simulink model "ident_2019b"  (R2019b)
settings: Solver=FixedStepAuto  StartTime=0.0  StopTime=20  FixedStep=Ts  RelTol=1e-3
values from neighbouring files (symbols this model uses):
  Flux = 0.00103001    [motor_parameters.sldd]
  Ld = 2.235E-5    [motor_parameters.sldd]
  Ls = 2.235E-5    [motor_parameters.sldd]
  Pn = 7.0    [motor_parameters.sldd]
  Rs = 0.112    [motor_parameters.sldd]
  Ts = 0.0001    [motor_parameters.sldd]
  Ubus = 12.0    [motor_parameters.sldd]
undefined symbols (not defined in the file or in its folder): magnitude
libraries: mcbplantlib x1, mcbcontrolslib x1, autolibpmsmexterior x1
settings Model: DataDictionary=motor_parameters.sldd  Creator=chenpeng  LastModifiedBy=ackict

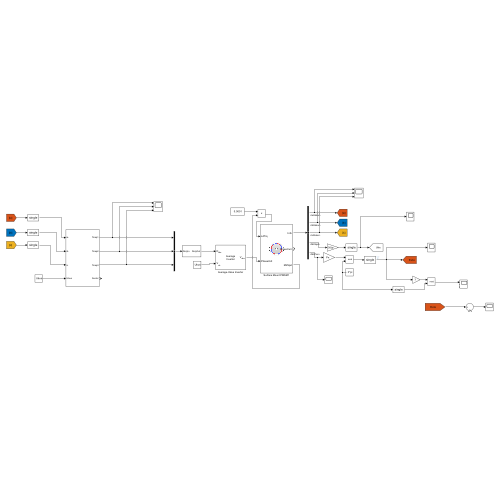
[thumbnail: Simulink's stored preview of the top-level diagram]
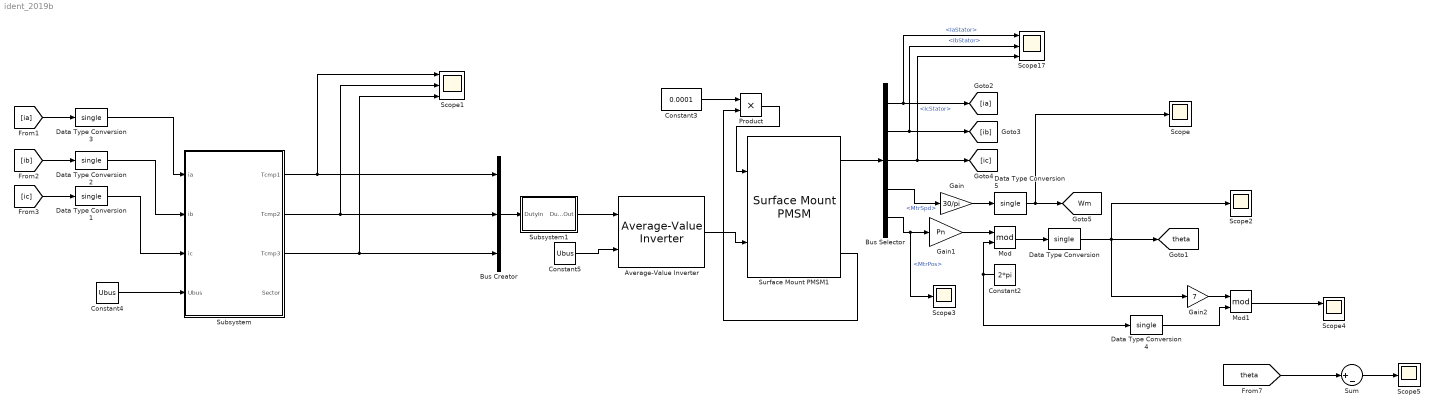
== system ident_2019b ==
  Average-Value Inverter : mcbplantlib/Average-Value Inverter
  Bus Creator : BusCreator  Inputs=3
  Bus Selector : BusSelector  OutputSignals=IaStator,IbStator,IcStator,MtrSpd,MtrPos
  Constant2 : Constant  Value=2*pi
  Constant3 : Constant  Value=0.0001  OutDataTypeStr=double
  Constant4 : Constant  Value=Ubus  OutDataTypeStr=single
  Constant5 : Constant  Value=Ubus  OutDataTypeStr=single
  Data Type Conversion{,1..5} (6 alike) : DataTypeConversion  OutDataTypeStr=single
  Gain : Gain  Gain=30/pi
  Gain1 : Gain  Gain=Pn
  Gain2 : Gain  Gain=7
  Mod : Math  Operator=mod  SaturateOnIntegerOverflow=on
  Mod1 : Math  Operator=mod  SaturateOnIntegerOverflow=on
  Product : Product
  Scope{,2..3,5} (4 alike) : Scope
  Scope1 : Scope  NumInputPorts=3
  Scope17 : Scope  NumInputPorts=3
  Scope4 : Scope  NumInputPorts=2
  Subsystem : Subsystem
  Subsystem1 : Subsystem
  Sum : Sum  Inputs=|+-
  Surface Mount PMSM1 : autolibpmsmexterior/Surface Mount PMSM  port_config=Torque  sim_type=Discrete  Ts=Ts  FilePath=E:\Sandbox\Bauto\Work\surfacepmsm_motordata.m  P=Pn  Rs=Rs  Ldq_=Ls  KConstText=Permanent flux linkage constant (lambda_pm):  lambda_pm=Flux  Ke=159.9771  Kt=1.323  mechanical=[0.0027, 4.924e-4, 0]  idq0=[0 0]  theta_init=0  omega_init=0  KConst=Flux  lambda_pm_calc=Flux  RefBlkName='autolibpmsmexterior/Surface Mount PMSM'  aMode=1  Ldq="[0.0003752   0.0003752]"
  tag scope: Wm=global, theta=global
  wires:
  Data Type Conversion3/1 -> Subsystem/1(ia)
  [ic] -> Data Type Conversion1/1
  Data Type Conversion1/1 -> Subsystem/3(ic)
  [ib] -> Data Type Conversion2/1
  [ia] -> Data Type Conversion3/1
  Data Type Conversion2/1 -> Subsystem/2(ib)
  Constant4/1 -> Subsystem/4(Ubus)
  Mod/1 -> Data Type Conversion/1
  Bus Selector/2 -> Scope17/2, [ib]  "<IbStator>"
  Subsystem/3(Tcmp3) -> Scope1/3, Bus Creator/3
  Data Type Conversion4/1 -> Mod1/2
  Constant2/1 -> Data Type Conversion4/1, Mod/2
  Subsystem/1(Tcmp1) -> Bus Creator/1, Scope1/1
  [theta] -> Sum/1
  Sum/1 -> Scope5/1
  Subsystem/2(Tcmp2) -> Scope1/2, Bus Creator/2
  Bus Selector/4 -> Gain/1  "<MtrSpd>"
  Product/1 -> Surface Mount PMSM1/1
  Mod1/1 -> Scope4/1
  Surface Mount PMSM1/1 -> Bus Selector/1
  Gain2/1 -> Mod1/1
  Surface Mount PMSM1/3 -> Product/2
  Subsystem1/1(DutyOut) -> Average-Value Inverter/1
  Constant5/1 -> Average-Value Inverter/2
  Average-Value Inverter/1 -> Surface Mount PMSM1/2
  Bus Selector/1 -> [ia], Scope17/1  "<IaStator>"
  Bus Selector/5 -> Scope3/1, Gain1/1  "<MtrPos>"
  Bus Creator/1 -> Subsystem1/1(DutyIn)
  Data Type Conversion/1 -> Scope2/1, Gain2/1, [theta]
  Bus Selector/3 -> Scope17/3, [ic]  "<IcStator>"
  Gain1/1 -> Mod/1
  Constant3/1 -> Product/1
  Data Type Conversion5/1 -> Scope/1, [Wm]
  Gain/1 -> Data Type Conversion5/1

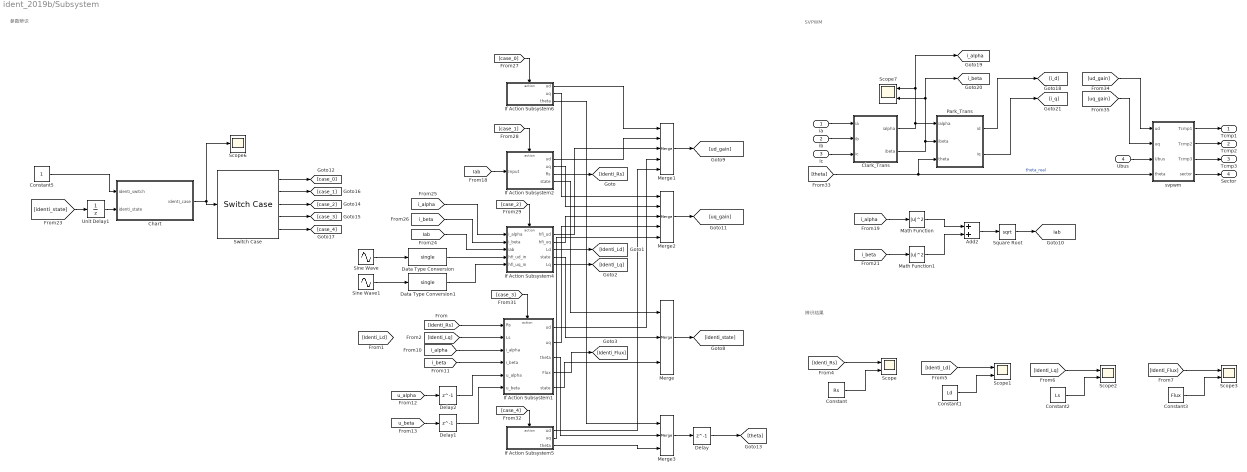
== system ident_2019b/Subsystem ==
  note: 参数辨识
  note: 辨识结果
  note: SVPWM
  ia : Inport  OutDataTypeStr=single  SampleTime=0.0001
  ib : Inport  Port=2  OutDataTypeStr=single  SampleTime=0.0001
  ic : Inport  Port=3  OutDataTypeStr=single  SampleTime=0.0001
  Ubus : Inport  Port=4  SampleTime=0.0001
  Add2 : Sum
  Chart : Stateflow chart  TreatAsAtomicUnit=on
  Clark_Trans : Subsystem  TreatAsAtomicUnit=on
  Constant : Constant  Value=Rs  OutDataTypeStr=single
  Constant1 : Constant  Value=Ld  OutDataTypeStr=single
  Constant2 : Constant  Value=Ls  OutDataTypeStr=single
  Constant3 : Constant  Value=Flux  OutDataTypeStr=single
  Constant5 : Constant  OutDataTypeStr=single
  Data Type Conversion : DataTypeConversion  OutDataTypeStr=single
  Data Type Conversion1 : DataTypeConversion  OutDataTypeStr=single
  Delay : Delay  DelayLength=1
  Delay1 : Delay  DelayLength=1
  Delay2 : Delay  DelayLength=1
  If Action Subsystem1 : Subsystem  TreatAsAtomicUnit=on
  If Action Subsystem2 : Subsystem  TreatAsAtomicUnit=on
  If Action Subsystem4 : Subsystem  TreatAsAtomicUnit=on
  If Action Subsystem5 : Subsystem  TreatAsAtomicUnit=on
  If Action Subsystem6 : Subsystem  TreatAsAtomicUnit=on
  Math Function : Math  Operator=magnitude^2  SignedPower=on  OutputSignalType=real  SaturateOnIntegerOverflow=on
  Math Function1 : Math  Operator=magnitude^2  SignedPower=on  OutputSignalType=real  SaturateOnIntegerOverflow=on
  Merge : Merge  Inputs=3
  Merge1 : Merge  Inputs=5
  Merge2 : Merge  Inputs=5
  Merge3 : Merge  Inputs=3
  Park_Trans : Subsystem  TreatAsAtomicUnit=on
  Scope{,1..3,7} (5 alike) : Scope  NumInputPorts=2
  Scope6 : Scope
  Sine Wave : Sin  Amplitude=2  Frequency=1884  SampleTime=0.0001
  Sine Wave1 : Sin  Amplitude=2  Frequency=1884  Phase=pi/2  SampleTime=0.0001
  Square Root : Sqrt  SaturateOnIntegerOverflow=on
  Switch Case : SwitchCase  CaseConditions={0,1,2,3,4}  ShowDefaultCase=off
  Unit Delay1 : UnitDelay  SampleTime=-1  HasFrameUpgradeWarning=on
  svpwm : Subsystem
  Tcmp1 : Outport
  Tcmp2 : Outport  Port=2
  Tcmp3 : Outport  Port=3
  Sector : Outport  Port=4
  tag scope: Iab=global, i_alpha=global, i_beta=global
  wires:
  If Action Subsystem6/1(ud) -> Merge1/1
  Data Type Conversion1/1 -> If Action Subsystem4/5(hfi_uq_in)
  Switch Case/1 -> [case_0]
  If Action Subsystem1/4(Flux) -> [Identi_Flux]
  If Action Subsystem4/2(hfi_uq) -> Merge2/3
  Merge/1 -> [identi_state]
  Ubus/1 -> svpwm/3(Ubus)
  Clark_Trans/2(ibeta) -> [i_beta], Scope7/2, Park_Trans/2(ibeta)
  If Action Subsystem4/4(state) -> Merge/2
  Switch Case/4 -> [case_3]
  If Action Subsystem2/2(uq) -> Merge2/2
  Clark_Trans/1(ialpha) -> [i_alpha], Scope7/1, Park_Trans/1(ialpha)
  Switch Case/2 -> [case_1]
  Merge3/1 -> Delay/1
  Math Function1/1 -> Add2/2
  [i_beta] -> If Action Subsystem4/2(i_beta)
  [theta] -> svpwm/4(theta), Park_Trans/3(theta)  "theta_real"
  [Iab] -> If Action Subsystem4/3(iab)
  If Action Subsystem6/3(theta) -> Merge3/1
  [ud_gain] -> svpwm/1(ud)
  Data Type Conversion/1 -> If Action Subsystem4/4(hfi_ud_in)
  If Action Subsystem5/2(uq) -> Merge2/5
  svpwm/4(sector) -> Sector/1
  Park_Trans/2(iq) -> [i_q]
  [case_3] -> If Action Subsystem1/Action
  Sine Wave/1 -> Data Type Conversion/1
  If Action Subsystem2/1(ud) -> Merge1/2
  Switch Case/3 -> [case_2]
  svpwm/1(Tcmp1) -> Tcmp1/1
  Constant5/1 -> Chart/1(identi_switch)
  [case_1] -> If Action Subsystem2/Action
  ia/1 -> Clark_Trans/1(ia)
  ic/1 -> Clark_Trans/3(ic)
  If Action Subsystem1/2(uq) -> Merge2/4
  [i_alpha] -> Math Function/1
  Math Function/1 -> Add2/1
  ib/1 -> Clark_Trans/2(ib)
  If Action Subsystem1/1(ud) -> Merge1/4
  If Action Subsystem5/3(theta) -> Merge3/3
  Square Root/1 -> [Iab]
  [case_4] -> If Action Subsystem5/Action
  Park_Trans/1(id) -> [i_d]
  Add2/1 -> Square Root/1
  [i_alpha] -> If Action Subsystem4/1(i_alpha)
  [Iab] -> If Action Subsystem2/1(Input)
  If Action Subsystem1/3(theta) -> Merge3/2
  Chart/1(identi_case) -> Scope6/1, Switch Case/1
  [case_0] -> If Action Subsystem6/Action
  [Identi_Lq] -> If Action Subsystem1/2(Ls)
  Switch Case/5 -> [case_4]
  [case_2] -> If Action Subsystem4/Action
  [i_beta] -> Math Function1/1
  Unit Delay1/1 -> Chart/2(identi_state)
  [identi_state] -> Unit Delay1/1
  Merge1/1 -> [ud_gain]
  Sine Wave1/1 -> Data Type Conversion1/1
  If Action Subsystem4/1(hfi_ud) -> Merge1/3
  svpwm/2(Tcmp2) -> Tcmp2/1
  svpwm/3(Tcmp3) -> Tcmp3/1
  Merge2/1 -> [uq_gain]
  If Action Subsystem5/1(ud) -> Merge1/5
  [uq_gain] -> svpwm/2(uq)
  If Action Subsystem2/4(state) -> Merge/1
  If Action Subsystem1/5(state) -> Merge/3
  If Action Subsystem6/2(uq) -> Merge2/1
  If Action Subsystem4/3(Ld) -> [Identi_Ld]
  [Identi_Rs] -> If Action Subsystem1/1(Rs)
  If Action Subsystem2/3(Rs) -> [Identi_Rs]
  [Identi_Rs] -> Scope/1
  Constant/1 -> Scope/2
  [Identi_Ld] -> Scope1/1
  Constant1/1 -> Scope1/2
  [Identi_Lq] -> Scope2/1
  Constant2/1 -> Scope2/2
  [Identi_Flux] -> Scope3/1
  Constant3/1 -> Scope3/2
  If Action Subsystem4/5(Lq) -> [Identi_Lq]
  [i_alpha] -> If Action Subsystem1/3(i_alpha)
  [i_beta] -> If Action Subsystem1/4(i_beta)
  Delay/1 -> [theta]
  Delay2/1 -> If Action Subsystem1/5(u_alpha)
  [u_alpha] -> Delay2/1
  [u_beta] -> Delay1/1
  Delay1/1 -> If Action Subsystem1/6(u_beta)

== system ident_2019b/Subsystem1 ==
  DutyIn : Inport
  Constant : Constant  Value=0.5  OutDataTypeStr=double  SampleTime=-1
  Gain : Gain  Gain=1/8000  ParamDataTypeStr=single
  Gain1 : Gain  Gain=-1
  Sum : Sum  Inputs=|+-
  Sum1 : Sum  Inputs=|++
  DutyOut : Outport
  wires:
  Sum/1 -> Gain1/1
  Constant/1 -> Sum1/2, Sum/2
  DutyIn/1 -> Gain/1
  Gain1/1 -> Sum1/1
  Sum1/1 -> DutyOut/1
  Gain/1 -> Sum/1

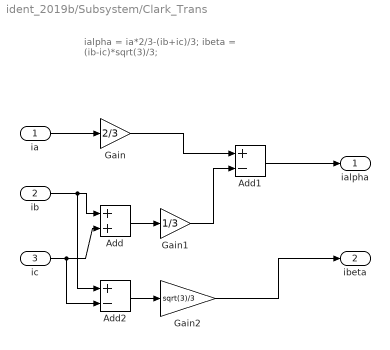
== system ident_2019b/Subsystem/Clark_Trans ==
  note: ialpha = ia*2/3-(ib+ic)/3;
      | ibeta = (ib-ic)*sqrt(3)/3;
  ia : Inport  OutDataTypeStr=single
  ib : Inport  Port=2  OutDataTypeStr=single
  ic : Inport  Port=3  OutDataTypeStr=single
  Add : Sum  AccumDataTypeStr=single  OutDataTypeStr=single
  Add1 : Sum  Inputs=+-  AccumDataTypeStr=single  OutDataTypeStr=single
  Add2 : Sum  Inputs=+-  AccumDataTypeStr=single  OutDataTypeStr=single
  Gain : Gain  Gain=2/3  ParamDataTypeStr=single
  Gain1 : Gain  Gain=1/3  ParamDataTypeStr=single
  Gain2 : Gain  Gain=sqrt(3)/3  ParamDataTypeStr=single
  ialpha : Outport  OutDataTypeStr=single
  ibeta : Outport  Port=2  OutDataTypeStr=single
  wires:
  ia/1 -> Gain/1
  ib/1 -> Add2/1, Add/1
  ic/1 -> Add2/2, Add/2
  Add/1 -> Gain1/1
  Gain/1 -> Add1/1
  Gain1/1 -> Add1/2
  Add1/1 -> ialpha/1
  Add2/1 -> Gain2/1
  Gain2/1 -> ibeta/1

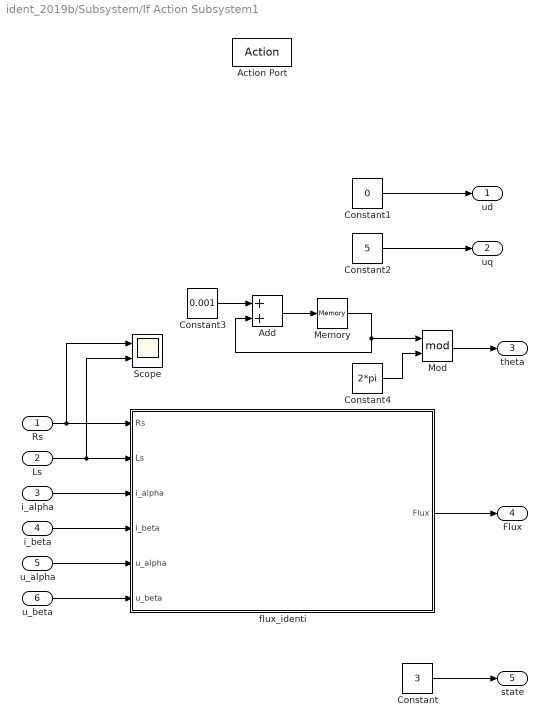
== system ident_2019b/Subsystem/If Action Subsystem1 ==
  Rs : Inport  OutDataTypeStr=single
  Ls : Inport  Port=2  OutDataTypeStr=single
  i_alpha : Inport  Port=3  OutDataTypeStr=single
  i_beta : Inport  Port=4  OutDataTypeStr=single
  u_alpha : Inport  Port=5  OutDataTypeStr=single
  u_beta : Inport  Port=6  OutDataTypeStr=single
  Action Port : ActionPort  ActionPortLabel=case [ 3 ]:
  Add : Sum
  Constant : Constant  Value=3  OutDataTypeStr=single
  Constant1 : Constant  Value=0  OutDataTypeStr=single
  Constant2 : Constant  Value=5  OutDataTypeStr=single
  Constant3 : Constant  Value=0.001  OutDataTypeStr=single
  Constant4 : Constant  Value=2*pi  OutDataTypeStr=single
  Memory : Memory
  Mod : Math  Operator=mod  SaturateOnIntegerOverflow=on
  Scope : Scope  NumInputPorts=2
  flux_identi : Subsystem
  ud : Outport  OutDataTypeStr=single
  uq : Outport  Port=2  OutDataTypeStr=single
  theta : Outport  Port=3  OutDataTypeStr=single
  Flux : Outport  Port=4  OutDataTypeStr=single
  state : Outport  Port=5  OutDataTypeStr=single
  wires:
  Constant/1 -> state/1
  Rs/1 -> Scope/1, flux_identi/1(Rs)
  Ls/1 -> Scope/2, flux_identi/2(Ls)
  flux_identi/1(Flux) -> Flux/1
  i_alpha/1 -> flux_identi/3(i_alpha)
  i_beta/1 -> flux_identi/4(i_beta)
  u_alpha/1 -> flux_identi/5(u_alpha)
  u_beta/1 -> flux_identi/6(u_beta)
  Constant1/1 -> ud/1
  Constant2/1 -> uq/1
  Constant3/1 -> Add/1
  Add/1 -> Memory/1
  Memory/1 -> Mod/1, Add/2
  Constant4/1 -> Mod/2
  Mod/1 -> theta/1

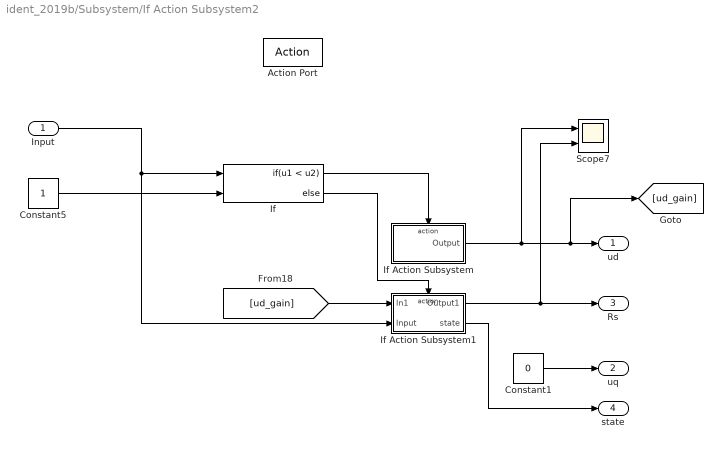
== system ident_2019b/Subsystem/If Action Subsystem2 ==
  Input : Inport  OutDataTypeStr=single
  Action Port : ActionPort  ActionPortLabel=case [ 1 ]:
  Constant1 : Constant  Value=0  OutDataTypeStr=single
  Constant5 : Constant  OutDataTypeStr=single
  If : If  NumInputs=2  IfExpression=u1 < u2
  If Action Subsystem : Subsystem  TreatAsAtomicUnit=on
  If Action Subsystem1 : Subsystem  TreatAsAtomicUnit=on
  Scope7 : Scope  NumInputPorts=2
  ud : Outport  OutDataTypeStr=single
  uq : Outport  Port=2  OutDataTypeStr=single
  Rs : Outport  Port=3  OutDataTypeStr=single
  state : Outport  Port=4  OutDataTypeStr=single
  wires:
  [ud_gain] -> If Action Subsystem1/1(In1)
  If/1 -> If Action Subsystem/Action
  If Action Subsystem/1(Output) -> Scope7/1, [ud_gain], ud/1
  Constant5/1 -> If/2
  If/2 -> If Action Subsystem1/Action
  Input/1 -> If Action Subsystem1/2(Input), If/1
  If Action Subsystem1/1(Output1) -> Rs/1, Scope7/2
  Constant1/1 -> uq/1
  If Action Subsystem1/2(state) -> state/1

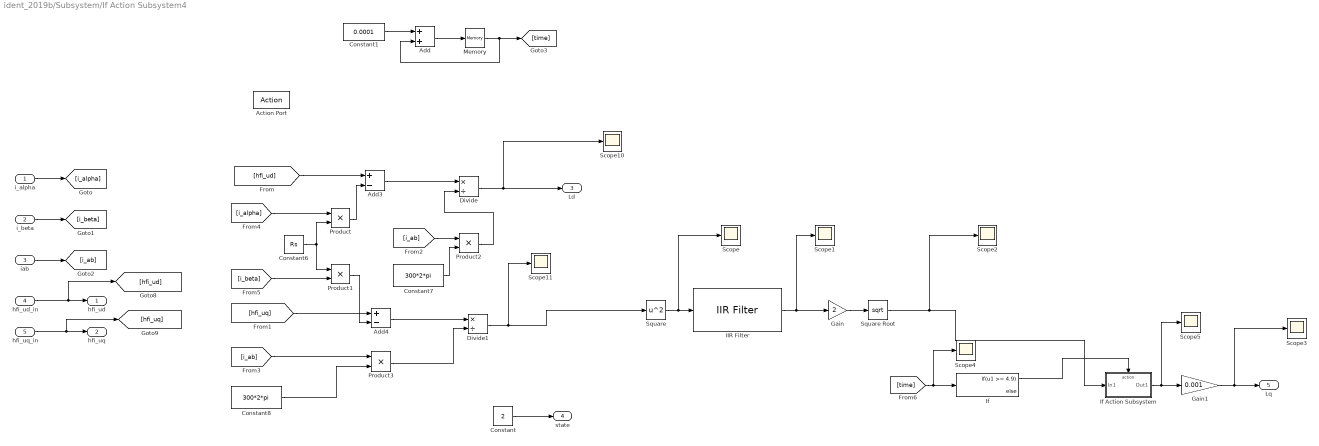
== system ident_2019b/Subsystem/If Action Subsystem4 ==
  i_alpha : Inport  OutDataTypeStr=single
  i_beta : Inport  Port=2  OutDataTypeStr=single
  iab : Inport  Port=3  OutDataTypeStr=single
  hfi_ud_in : Inport  Port=4  OutDataTypeStr=single
  hfi_uq_in : Inport  Port=5  OutDataTypeStr=single
  Action Port : ActionPort  ActionPortLabel=case [ 2 ]:
  Add : Sum
  Add3 : Sum  Inputs=+-  OutDataTypeStr=single
  Add4 : Sum  Inputs=+-  OutDataTypeStr=single
  Constant : Constant  Value=2  OutDataTypeStr=single
  Constant1 : Constant  Value=0.0001  OutDataTypeStr=single
  Constant6 : Constant  Value=Rs  OutDataTypeStr=single
  Constant7 : Constant  Value=300*2*pi  OutDataTypeStr=single
  Constant8 : Constant  Value=300*2*pi  OutDataTypeStr=single
  Divide : Product  Inputs=*/  OutDataTypeStr=single
  Divide1 : Product  Inputs=*/
  Gain : Gain  Gain=2
  Gain1 : Gain  Gain=0.001
  IIR Filter : mcbcontrolslib/IIR Filter  VariantControl=Low Pass Filter  VariantSelect=Low-pass  Filter_constant=0.0063  advancedSettings=on  Ts=1e-4  cutOff_freq=10.0903
  If : If  IfExpression=u1 >= 4.9
  If Action Subsystem : Subsystem  TreatAsAtomicUnit=on
  Memory : Memory
  Product : Product  OutDataTypeStr=single
  Product1 : Product  OutDataTypeStr=single
  Product2 : Product  OutDataTypeStr=single
  Product3 : Product
  Scope{,1..5,10..11} (8 alike) : Scope
  Square : Math  Operator=square  SaturateOnIntegerOverflow=on
  Square Root : Sqrt  OutDataTypeStr=single  SaturateOnIntegerOverflow=on
  hfi_ud : Outport  OutDataTypeStr=single
  hfi_uq : Outport  Port=2  OutDataTypeStr=single
  Ld : Outport  Port=3  OutDataTypeStr=single
  state : Outport  Port=4  OutDataTypeStr=single
  Lq : Outport  Port=5  OutDataTypeStr=single
  wires:
  Product/1 -> Add3/2
  Constant8/1 -> Product3/2
  Product3/1 -> Divide1/2
  Divide1/1 -> Square/1, Scope11/1
  [i_ab] -> Product3/1
  [hfi_uq] -> Add4/1
  Divide/1 -> Ld/1, Scope10/1
  [i_ab] -> Product2/1
  Product1/1 -> Add4/2
  Product2/1 -> Divide/2
  Add4/1 -> Divide1/1
  Constant7/1 -> Product2/2
  [hfi_ud] -> Add3/1
  Constant6/1 -> Product1/1, Product/2
  Add3/1 -> Divide/1
  [i_beta] -> Product1/2
  [i_alpha] -> Product/1
  Constant/1 -> state/1
  i_alpha/1 -> [i_alpha]
  i_beta/1 -> [i_beta]
  iab/1 -> [i_ab]
  hfi_uq_in/1 -> [hfi_uq], hfi_uq/1
  hfi_ud_in/1 -> [hfi_ud], hfi_ud/1
  Gain/1 -> Square Root/1
  Square/1 -> Scope/1, IIR Filter/1
  IIR Filter/1 -> Scope1/1, Gain/1
  Square Root/1 -> Scope2/1, If Action Subsystem/1(In1)
  Constant1/1 -> Add/1
  Add/1 -> Memory/1
  Memory/1 -> Add/2, [time]
  [time] -> Scope4/1, If/1
  If/1 -> If Action Subsystem/Action
  If Action Subsystem/1(Out1) -> Scope5/1, Gain1/1
  Gain1/1 -> Lq/1, Scope3/1

== system ident_2019b/Subsystem/If Action Subsystem5 ==
  Action Port : ActionPort  ActionPortLabel=case [ 4 ]:
  Constant : Constant  Value=0  OutDataTypeStr=single
  Constant1 : Constant  Value=0  OutDataTypeStr=single
  Constant2 : Constant  Value=0  OutDataTypeStr=single
  ud : Outport
  uq : Outport  Port=2  OutDataTypeStr=single
  theta : Outport  Port=3
  wires:
  Constant/1 -> uq/1
  Constant1/1 -> ud/1
  Constant2/1 -> theta/1

== system ident_2019b/Subsystem/If Action Subsystem6 ==
  Action Port : ActionPort  ActionPortLabel=case [ 0 ]:
  Constant : Constant  Value=0  OutDataTypeStr=single
  Constant1 : Constant  Value=0  OutDataTypeStr=single
  Constant2 : Constant  Value=0  OutDataTypeStr=single
  ud : Outport
  uq : Outport  Port=2  OutDataTypeStr=single
  theta : Outport  Port=3
  wires:
  Constant2/1 -> theta/1
  Constant1/1 -> ud/1
  Constant/1 -> uq/1

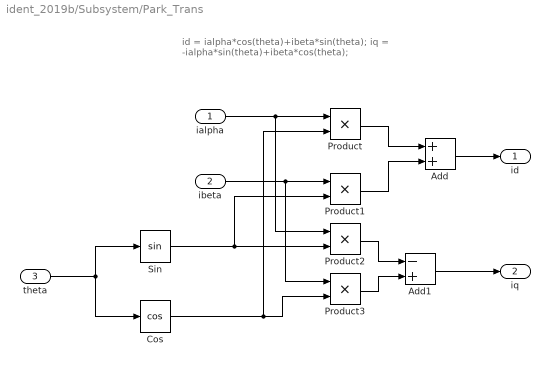
== system ident_2019b/Subsystem/Park_Trans ==
  note: id = ialpha*cos(theta)+ibeta*sin(theta);
      | iq = -ialpha*sin(theta)+ibeta*cos(theta);
  ialpha : Inport  OutDataTypeStr=single
  ibeta : Inport  Port=2  OutDataTypeStr=single
  theta : Inport  Port=3  OutDataTypeStr=single
  Add : Sum  AccumDataTypeStr=single  OutDataTypeStr=single
  Add1 : Sum  Inputs=-+  AccumDataTypeStr=single  OutDataTypeStr=single
  Cos : Trigonometry  Operator=cos  ApproximationMethod=CORDIC
  Product{,1..3} (4 alike) : Product  OutDataTypeStr=single
  Sin : Trigonometry  ApproximationMethod=CORDIC
  id : Outport  OutDataTypeStr=single
  iq : Outport  Port=2  OutDataTypeStr=single
  wires:
  ialpha/1 -> Product2/1, Product/1
  ibeta/1 -> Product3/1, Product1/1
  Product/1 -> Add/1
  Product1/1 -> Add/2
  Add/1 -> id/1
  Product2/1 -> Add1/1
  Product3/1 -> Add1/2
  Add1/1 -> iq/1
  theta/1 -> Cos/1, Sin/1
  Sin/1 -> Product1/2, Product2/2
  Cos/1 -> Product/2, Product3/2

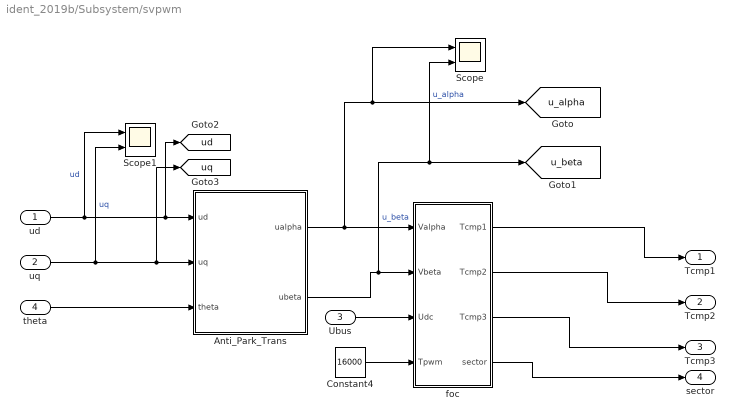
== system ident_2019b/Subsystem/svpwm ==
  ud : Inport  OutDataTypeStr=single
  uq : Inport  Port=2
  Ubus : Inport  Port=3  SampleTime=0.0001
  theta : Inport  Port=4
  Anti_Park_Trans : Subsystem  TreatAsAtomicUnit=on
  Constant4 : Constant  Value=16000  OutDataTypeStr=single
  Scope : Scope  NumInputPorts=2
  Scope1 : Scope  NumInputPorts=2
  foc : MATLAB Function  TreatAsAtomicUnit=on
  Tcmp1 : Outport
  Tcmp2 : Outport  Port=2
  Tcmp3 : Outport  Port=3
  sector : Outport  Port=4
  tag scope: u_alpha=global, u_beta=global, ud=global, uq=global
  wires:
  foc/1(Tcmp1) -> Tcmp1/1
  Constant4/1 -> foc/4(Tpwm)
  Ubus/1 -> foc/3(Udc)
  uq/1 -> Scope1/2, [uq], Anti_Park_Trans/2(uq)  "uq"
  foc/4(sector) -> sector/1
  ud/1 -> Scope1/1, [ud], Anti_Park_Trans/1(ud)  "ud"
  foc/3(Tcmp3) -> Tcmp3/1
  foc/2(Tcmp2) -> Tcmp2/1
  theta/1 -> Anti_Park_Trans/3(theta)
  Anti_Park_Trans/1(ualpha) -> Scope/1, [u_alpha], foc/1(Valpha)  "u_alpha"
  Anti_Park_Trans/2(ubeta) -> Scope/2, [u_beta], foc/2(Vbeta)  "u_beta"

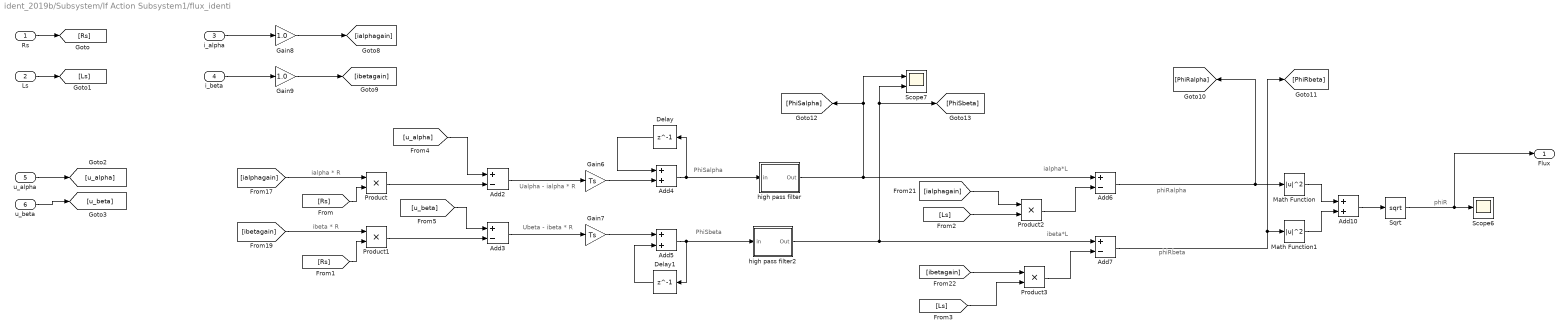
== system ident_2019b/Subsystem/If Action Subsystem1/flux_identi ==
  note: phiRbeta
  note: phiR
  note: ialpha * R
  note: PhiSbeta
  note: phiRalpha
  note: ialpha*L
  note: ibeta * R
  note: Ubeta - ibeta * R
  note: Ualpha - ialpha * R
  note: PhiSalpha
  note: ibeta*L
  Rs : Inport  OutDataTypeStr=single
  Ls : Inport  Port=2  OutDataTypeStr=single
  i_alpha : Inport  Port=3  OutDataTypeStr=single
  i_beta : Inport  Port=4  OutDataTypeStr=single
  u_alpha : Inport  Port=5  OutDataTypeStr=single
  u_beta : Inport  Port=6  OutDataTypeStr=single
  Add10 : Sum
  Add{2..3,6..7} (4 alike) : Sum  Inputs=+-
  Add4 : Sum
  Add5 : Sum
  Delay : Delay  DelayLength=1  InitialCondition=0
  Delay1 : Delay  DelayLength=1
  Gain6 : Gain  Gain=Ts
  Gain7 : Gain  Gain=Ts
  Gain8 : Gain  Gain=1.0
  Gain9 : Gain  Gain=1.0
  Math Function : Math  Operator=magnitude^2  SignedPower=on  OutputSignalType=real  SaturateOnIntegerOverflow=on
  Math Function1 : Math  Operator=magnitude^2  SignedPower=on  OutputSignalType=real  SaturateOnIntegerOverflow=on
  Product{,1..3} (4 alike) : Product
  Scope6 : Scope
  Scope7 : Scope  NumInputPorts=2
  Sqrt : Sqrt  SaturateOnIntegerOverflow=on
  high pass filter : Subsystem  mask{fc=10, Ts=Ts}
      mask prompts: fc "cut off freq"; Ts "simple rate"
      mask help: High pass filter
  high pass filter2 : Subsystem  mask{fc=10, Ts=Ts}
      mask prompts: fc "cut off freq"; Ts "simple rate"
      mask help: High pass filter
  Flux : Outport  OutDataTypeStr=single
  wires:
  Math Function1/1 -> Add10/2
  [u_beta] -> Add3/1
  Add6/1 -> [PhiRalpha], Math Function/1
  Add3/1 -> Gain7/1
  [ibetagain] -> Product3/1
  Add5/1 -> Delay1/1, high pass filter2/1(in)
  Add4/1 -> Delay/1, high pass filter/1(in)
  high pass filter/1(Out) -> [PhiSalpha], Scope7/1, Add6/1
  Gain6/1 -> Add4/2
  [ibetagain] -> Product1/1
  Add10/1 -> Sqrt/1
  Delay1/1 -> Add5/2
  [ialphagain] -> Product/1
  Math Function/1 -> Add10/1
  [u_alpha] -> Add2/1
  Product/1 -> Add2/2
  Product3/1 -> Add7/2
  Delay/1 -> Add4/1
  Add2/1 -> Gain6/1
  Sqrt/1 -> Flux/1, Scope6/1
  Product1/1 -> Add3/2
  i_beta/1 -> Gain9/1
  Add7/1 -> [PhiRbeta], Math Function1/1
  Gain7/1 -> Add5/1
  i_alpha/1 -> Gain8/1
  high pass filter2/1(Out) -> [PhiSbeta], Scope7/2, Add7/1
  Gain9/1 -> [ibetagain]
  Gain8/1 -> [ialphagain]
  Rs/1 -> [Rs]
  Ls/1 -> [Ls]
  [Rs] -> Product/2
  [Rs] -> Product1/2
  [ialphagain] -> Product2/1
  Product2/1 -> Add6/2
  [Ls] -> Product2/2
  [Ls] -> Product3/2
  u_alpha/1 -> [u_alpha]
  u_beta/1 -> [u_beta]

== system ident_2019b/Subsystem/If Action Subsystem2/If Action Subsystem ==
  Action Port : ActionPort  ActionPortLabel=if(u1 < u2)
  Add3 : Sum
  Constant6 : Constant  Value=0.01  OutDataTypeStr=single
  Memory : Memory  InheritSampleTime=on
  Output : Outport  OutDataTypeStr=single
  wires:
  Memory/1 -> Output/1, Add3/2
  Add3/1 -> Memory/1
  Constant6/1 -> Add3/1

== system ident_2019b/Subsystem/If Action Subsystem2/If Action Subsystem1 ==
  In1 : Inport  OutDataTypeStr=single
  Input : Inport  Port=2  OutDataTypeStr=single
  Action Port : ActionPort  ActionPortLabel=else
  Constant : Constant  OutDataTypeStr=single
  Divide : Product  Inputs=*/
  Output1 : Outport  OutDataTypeStr=single
  state : Outport  Port=2  OutDataTypeStr=single
  wires:
  In1/1 -> Divide/1
  Input/1 -> Divide/2
  Divide/1 -> Output1/1
  Constant/1 -> state/1

== system ident_2019b/Subsystem/If Action Subsystem4/If Action Subsystem ==
  In1 : Inport  OutDataTypeStr=single
  Action Port : ActionPort  ActionPortLabel=if(u1 >= 4.9)
  Memory : Memory
  Scope : Scope
  Sum : Sum  Inputs=|++
  Out1 : Outport  OutDataTypeStr=single
  wires:
  In1/1 -> Scope/1, Sum/1
  Sum/1 -> Memory/1
  Memory/1 -> Out1/1, Sum/2

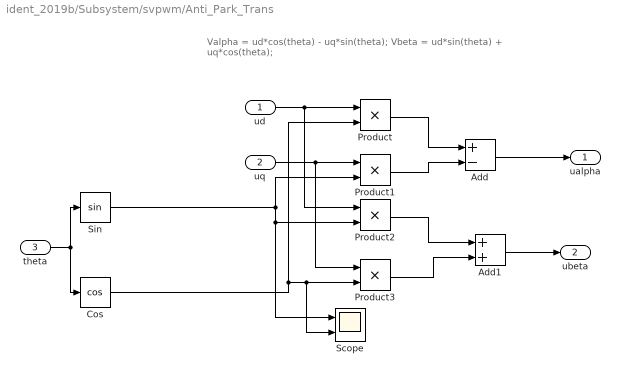
== system ident_2019b/Subsystem/svpwm/Anti_Park_Trans ==
  note: Valpha = ud*cos(theta) - uq*sin(theta);
      | Vbeta = ud*sin(theta) + uq*cos(theta);
  ud : Inport  OutDataTypeStr=single
  uq : Inport  Port=2  OutDataTypeStr=single
  theta : Inport  Port=3
  Add : Sum  Inputs=+-
  Add1 : Sum
  Cos : Trigonometry  Operator=cos
  Product{,1..3} (4 alike) : Product
  Scope : Scope  NumInputPorts=2
  Sin : Trigonometry
  ualpha : Outport  OutDataTypeStr=single
  ubeta : Outport  Port=2  OutDataTypeStr=single
  wires:
  Add/1 -> ualpha/1
  ud/1 -> Product2/1, Product/1
  Cos/1 -> Product/2, Scope/2, Product3/2
  Product/1 -> Add/1
  uq/1 -> Product3/1, Product1/1
  theta/1 -> Sin/1, Cos/1
  Product1/1 -> Add/2
  Product2/1 -> Add1/1
  Product3/1 -> Add1/2
  Add1/1 -> ubeta/1
  Sin/1 -> Scope/1, Product2/2, Product1/2

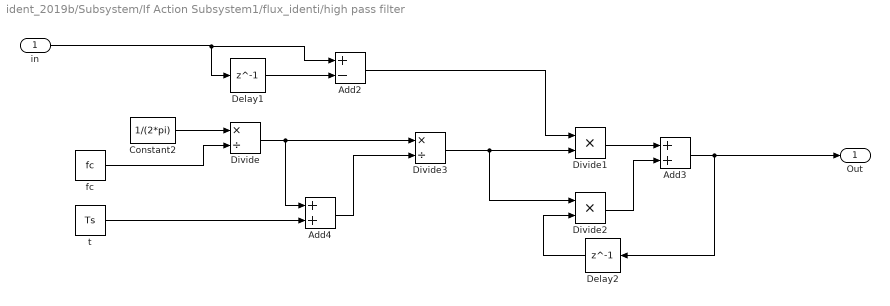
== system ident_2019b/Subsystem/If Action Subsystem1/flux_identi/high pass filter ==
  in : Inport
  Add2 : Sum  Inputs=+-
  Add3 : Sum
  Add4 : Sum
  Constant2 : Constant  Value=1/(2*pi)  OutDataTypeStr=single
  Delay1 : Delay  DelayLength=1
  Delay2 : Delay  DelayLength=1
  Divide : Product  Inputs=*/
  Divide1 : Product  Inputs=**
  Divide2 : Product  Inputs=**
  Divide3 : Product  Inputs=*/
  fc : Constant  Value=fc  OutDataTypeStr=single
  t : Constant  Value=Ts  OutDataTypeStr=single
  Out : Outport
  wires:
  Divide/1 -> Add4/1, Divide3/1
  Divide2/1 -> Add3/2
  Add3/1 -> Out/1, Delay2/1
  Divide3/1 -> Divide2/1, Divide1/2
  Add2/1 -> Divide1/1
  in/1 -> Add2/1, Delay1/1
  t/1 -> Add4/2
  Divide1/1 -> Add3/1
  Add4/1 -> Divide3/2
  fc/1 -> Divide/2
  Delay2/1 -> Divide2/2
  Delay1/1 -> Add2/2
  Constant2/1 -> Divide/1

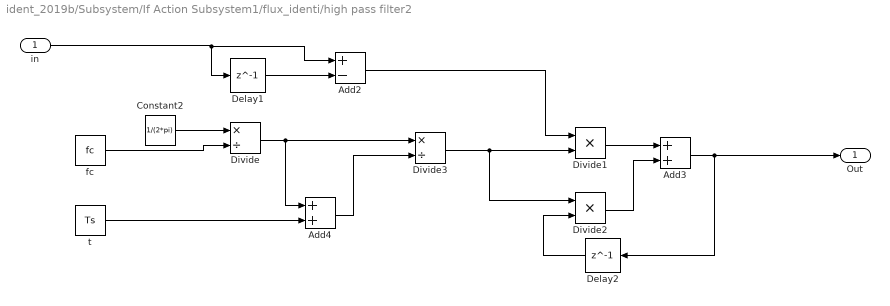
== system ident_2019b/Subsystem/If Action Subsystem1/flux_identi/high pass filter2 ==
  in : Inport
  Add2 : Sum  Inputs=+-
  Add3 : Sum
  Add4 : Sum
  Constant2 : Constant  Value=1/(2*pi)  OutDataTypeStr=single
  Delay1 : Delay  DelayLength=1
  Delay2 : Delay  DelayLength=1
  Divide : Product  Inputs=*/
  Divide1 : Product  Inputs=**
  Divide2 : Product  Inputs=**
  Divide3 : Product  Inputs=*/
  fc : Constant  Value=fc  OutDataTypeStr=single
  t : Constant  Value=Ts  OutDataTypeStr=single
  Out : Outport
  wires:
  Constant2/1 -> Divide/1
  Delay1/1 -> Add2/2
  Delay2/1 -> Divide2/2
  fc/1 -> Divide/2
  Add4/1 -> Divide3/2
  Divide1/1 -> Add3/1
  t/1 -> Add4/2
  in/1 -> Delay1/1, Add2/1
  Add2/1 -> Divide1/1
  Divide3/1 -> Divide1/2, Divide2/1
  Add3/1 -> Delay2/1, Out/1
  Divide2/1 -> Add3/2
  Divide/1 -> Divide3/1, Add4/1

== stateflow chart ident_2019b/Subsystem/Chart ==
  state IDLE
    identi_case=0;
  state Rs_Identi
    identi_case=1;
  state Ls_Identi
    identi_case=2;
  state Flux_Identi
    identi_case=3;
  state Identi_Over
    identi_case=4;
  (default) -> IDLE
  Flux_Identi -> Identi_Over [order 2] : [after(10,sec)&&identi_state==3]
  IDLE -> Rs_Identi : [identi_switch==1]
  Ls_Identi -> Flux_Identi [order 2] : [after(5,sec)&&identi_state==2]
  Rs_Identi -> Ls_Identi [order 2] : [after(1,sec)&&identi_state==1]
  Rs_Identi -> IDLE [order 1] : [identi_switch==0]
  Ls_Identi -> IDLE [order 1] : [identi_switch==0]
  Flux_Identi -> IDLE [order 1] : [identi_switch==0]
  Identi_Over -> IDLE : [identi_switch==0]
  data: identi_switch input; identi_state input; identi_case output single

== matlab function ident_2019b/Subsystem/svpwm/foc ==
  data: Valpha input; Tcmp1 output; Vbeta input; Udc input; Tpwm input; Tcmp2 output; Tcmp3 output; sector output
function [Tcmp1,Tcmp2,Tcmp3,sector] = fcn(Valpha,Vbeta,Udc,Tpwm)
%#codegen

sector = single(0);
Tcmp1 = single(0);
Tcmp2 = single(0);
Tcmp3 = single(0);

%========Parameters statement================

    Vref1 = Vbeta;							                   
    Vref2 = (sqrt(3)*Valpha - Vbeta)/2; 				    
    Vref3 = (-sqrt(3)*Valpha - Vbeta)/2;					
   
 %========Sector calculation=================

  if (Vref1>0)
	   sector = single(1);
  end
  if (Vref2>0)
	   sector = sector+single(2);
  end
  if (Vref3>0)
       sector = sector+single(4);
  end

%======== X Y Z calculation===================

X = sqrt(3)*Vbeta*Tpwm/Udc;
Y = Tpwm/Udc*(3/2*Valpha+sqrt(3)/2*Vbeta);
Z = Tpwm/Udc*(-3/2*Valpha+sqrt(3)/2*Vbeta);	         

%==========Duty ratio calculation================
switch (sector)   
    case 1
        T1 = Z; T2 = Y; 
	case 2
        T1 = Y; T2 = -X; 
	case 3
        T1 = -Z; T2 = X; 
	case 4
        T1 = -X; T2 = Z;
	case 5
        T1 = X; T2 = -Y;
    otherwise
        T1 = -Y; T2 = -Z;
end

if T1+T2 > Tpwm
    T1 = T1/(T1+T2);
    T2 = T2/(T1+T2);
else
    T1 = T1;
    T2 = T2;
end
ta = (Tpwm-(T1+T2))/4.0;
tb = ta+T1/2;
tc = tb+T2/2;

%==========Duty ratio calculation================
switch (sector)
    case 1 
        Tcmp1=tb;
        Tcmp2=ta;
        Tcmp3=tc; 
        
    case 2 
        Tcmp1=ta;
        Tcmp2=tc;
        Tcmp3=tb; 
       
    case 3 
        Tcmp1=ta;
        Tcmp2=tb;
        Tcmp3=tc; 
        
    case 4 
        Tcmp1=tc;
        Tcmp2=tb;
        Tcmp3=ta;
        
    case 5 
        Tcmp1=tc;
        Tcmp2=ta;
        Tcmp3=tb;
        
   case 6
       Tcmp1=tb;
       Tcmp2=tc;
       Tcmp3=ta;
end
end
